simulink model "testbench_state2"  (R2015a)
settings: Solver=ode3  StartTime=0.0  StopTime=inf  RelTol=1e-3
libraries: legoev3lib x4
settings Model: SimulationMode=external  ExtModeTrigDuration=2  Creator=USER  LastModifiedBy=USER
settings OptimizationCC: OptimizeModelRefInitCode=on  LifeSpan=1
settings DebuggingCC: UnderspecifiedInitializationDetection=Classic  MergeDetectMultiDrivingBlocksExec=none
settings HardwareCC: ProdLargestAtomicInteger=Long  ProdLargestAtomicFloat=Float  ProdEndianess=LittleEndian  ProdHWDeviceType=ARM Compatible->ARM 9
settings RTWCC: SystemTargetFile=realtime.tlc  GenerateMakefile=off  TemplateMakefile=realtime.tmf  Description=Run on Target Hardware  RTWVerbose=off
settings ERTTargetCC: CombineOutputUpdateFcns=off  ERTSrcFileBannerTemplate=realtime_code_template.cgt  ERTHdrFileBannerTemplate=realtime_code_template.cgt  ERTDataSrcFileTemplate=realtime_code_template.cgt  ERTDataHdrFileTemplate=realtime_code_template.cgt  ERTCustomFileTemplate=realtime_file_process.tlc

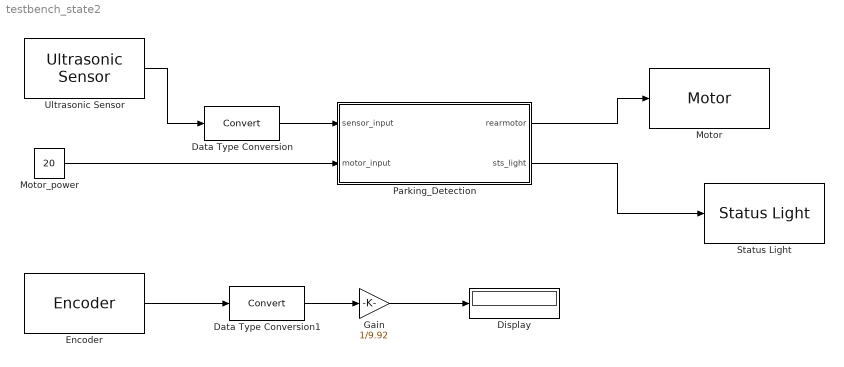
== system testbench_state2 ==
  Data Type Conversion : DataTypeConversion
  Data Type Conversion1 : DataTypeConversion
  Display : Display
  Encoder : legoev3lib/Encoder  portNumber=A  opMode=No reset  sampleTime=0.1
  Gain : Gain  Gain=1/9.92
  Motor : legoev3lib/Motor  sportNumber=A  sstopAction=Brake
  Motor_power : Constant  Value=20
  Parking_Detection : MATLAB Function  TreatAsAtomicUnit=on
  Status Light : legoev3lib/Status Light
  Ultrasonic Sensor : legoev3lib/Ultrasonic Sensor  PortNumber=1  sampleTime=0.1
  wires:
  Parking_Detection/1(rearmotor) -> Motor/1
  Parking_Detection/2(sts_light) -> Status Light/1
  Motor_power/1 -> Parking_Detection/2(motor_input)
  Ultrasonic Sensor/1 -> Data Type Conversion/1
  Data Type Conversion/1 -> Parking_Detection/1(sensor_input)
  Encoder/1 -> Data Type Conversion1/1
  Data Type Conversion1/1 -> Gain/1
  Gain/1 -> Display/1

== matlab function testbench_state2/Parking_Detection ==
  data: sensor_input input; rearmotor output; motor_input input; sts_light output
function [rearmotor,sts_light] = fcn(sensor_input,motor_input)
%#codegen
if(sensor_input>24)&&(sensor_input<=40)
   rearmotor=motor_input;
   sts_light=1;
else
   rearmotor=motor_input;
   sts_light=2;
end
end
